simulink library "calcAeroCoeffs_cl"  (R2020a)
settings: Solver=VariableStepAuto  StartTime=0.0  StopTime=10.0  RelTol=1e-3
libraries: calculateCXorCZorCM_ul x3, calculateCYorCLorCN_ul x3
settings Model: Creator=Ayaz  LastModifiedBy=Ayaz

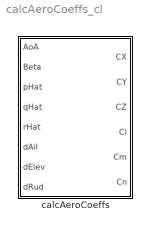
== system calcAeroCoeffs_cl ==
  calcAeroCoeffs : Subsystem  mask{C_X_AoA_coeffs=[8.32,0], C_X_qHat_coeffs=[4.41,-.6], C_X_dElev_coeffs=[0.11,-.01], C_X_0=0.46, C_Y_Beta_coeffs=-0.19, C_Y_pHat_coeffs=-0.1, C_Y_rHat_coeffs=[0.14,0.17], C_Y_dAil_coeffs=-0.05, C_Y_dRud_coeffs=0.1, C_Z_AoA_coeffs=[10.2,1.23,0], C_Z_qHat_coeffs=[6.15,0.13,-7.56], C_Z_dElev_coeffs=[0.29,0,-0.32], C_Z_0=-5.4, C_l_Beta_coeffs=-0.06, C_l_pHat_coeffs=-0.56, C_l_rHat_coeffs=[0.65,0.18], C_l_dAil_coeffs=[0.04,-0.25], C_l_dRud_coeffs=0, C_m_AoA_coeffs=[0.21,0], C_m_qHat_coeffs=[5.29,0,-11.30], C_m_dElev_coeffs=-1.02, C_m_0=-0.32, C_n_Beta_coeffs=[-0.09,0.06], C_n_pHat_coeffs=[-0.91,-0.06], C_n_rHat_coeffs=-0.05, C_n_dAil_coeffs=[-0.12,0.02], C_n_dRud_coeffs=-.04}
      mask prompts: C_X_AoA_coeffs "C_X_AoA polynomial coefficients (c0,c1,c2):"; C_X_qHat_coeffs "C_X_qHat polynomial coefficients (c0,c1,c2):"; C_X_dElev_coeffs "C_X_dElev polynomial coefficients (c0,c1,c2):"; C_X_0 "C_X_0 value"; C_Y_Beta_coeffs "C_Y_Beta polynomial coefficients (c0,c1,c2):"; C_Y_pHat_coeffs "C_Y_pHat polynomial coefficients (c0,c1,c2):"; C_Y_rHat_coeffs "C_Y_rHat polynomial coefficients (c0,c1,c2):"; C_Y_dAil_coeffs "C_Y_dAil polynomial coefficients (c0,c1,c2):"; C_Y_dRud_coeffs "C_Y_dRud polynomial coefficients (c0,c1,c2):"; C_Z_AoA_coeffs "C_Z_AoA polynomial coefficients (c0,c1,c2):"; C_Z_qHat_coeffs "C_Z_qHat polynomial coefficients (c0,c1,c2):"; C_Z_dElev_coeffs "C_Z_dElev polynomial coefficients (c0,c1,c2):"; C_Z_0 "C_Z_0 value"; C_l_Beta_coeffs "C_l_Beta polynomial coefficients (c0,c1,c2):"; C_l_pHat_coeffs "C_l_pHat polynomial coefficients (c0,c1,c2):"; C_l_rHat_coeffs "C_l_rHat polynomial coefficients (c0,c1,c2):"; C_l_dAil_coeffs "C_l_dAil polynomial coefficients (c0,c1,c2):"; C_l_dRud_coeffs "C_l_dRud polynomial coefficients (c0,c1,c2):"; C_m_AoA_coeffs "C_m_AoA polynomial coefficients (c0,c1,c2):"; C_m_qHat_coeffs "C_m_qHat polynomial coefficients (c0,c1,c2):"; C_m_dElev_coeffs "C_m_dElev polynomial coefficients (c0,c1,c2):"; C_m_0 "C_m_0 value"; C_n_Beta_coeffs "C_n_Beta polynomial coefficients (c0,c1,c2):"; C_n_pHat_coeffs "C_n_pHat polynomial coefficients (c0,c1,c2):"; C_n_rHat_coeffs "C_n_rHat polynomial coefficients (c0,c1,c2):"; C_n_dAil_coeffs "C_n_dAil polynomial coefficients (c0,c1,c2):"; C_n_dRud_coeffs "C_n_dRud polynomial coefficients (c0,c1,c2):"
      mask TypeOptions C_X_AoA_coeffs: calcCX/C_i_AoA_coeffs
      mask TypeOptions C_X_qHat_coeffs: calcCX/C_i_qHat_coeffs
      mask TypeOptions C_X_dElev_coeffs: calcCX/C_i_dElev_coeffs
      mask TypeOptions C_X_0: calcCX/C_i_0
      mask TypeOptions C_Y_Beta_coeffs: calcCY/C_i_Beta_coeffs
      mask TypeOptions C_Y_pHat_coeffs: calcCY/C_i_pHat_coeffs
      mask TypeOptions C_Y_rHat_coeffs: calcCY/C_i_rHat_coeffs
      mask TypeOptions C_Y_dAil_coeffs: calcCY/C_i_dAil_coeffs
      mask TypeOptions C_Y_dRud_coeffs: calcCY/C_i_dRud_coeffs
      mask TypeOptions C_Z_AoA_coeffs: calcCZ/C_i_AoA_coeffs
      mask TypeOptions C_Z_qHat_coeffs: calcCZ/C_i_qHat_coeffs
      mask TypeOptions C_Z_dElev_coeffs: calcCZ/C_i_dElev_coeffs
      mask TypeOptions C_Z_0: calcCZ/C_i_0
      mask TypeOptions C_l_Beta_coeffs: calcCl/C_i_Beta_coeffs
      mask TypeOptions C_l_pHat_coeffs: calcCl/C_i_pHat_coeffs
      mask TypeOptions C_l_rHat_coeffs: calcCl/C_i_rHat_coeffs
      mask TypeOptions C_l_dAil_coeffs: calcCl/C_i_dAil_coeffs
      mask TypeOptions C_l_dRud_coeffs: calcCl/C_i_dRud_coeffs
      mask TypeOptions C_m_AoA_coeffs: calcCm/C_i_AoA_coeffs
      mask TypeOptions C_m_qHat_coeffs: calcCm/C_i_qHat_coeffs
      mask TypeOptions C_m_dElev_coeffs: calcCm/C_i_dElev_coeffs
      mask TypeOptions C_m_0: calcCm/C_i_0
      mask TypeOptions C_n_Beta_coeffs: calcCn/C_i_Beta_coeffs
      mask TypeOptions C_n_pHat_coeffs: calcCn/C_i_pHat_coeffs
      mask TypeOptions C_n_rHat_coeffs: calcCn/C_i_rHat_coeffs
      mask TypeOptions C_n_dAil_coeffs: calcCn/C_i_dAil_coeffs
      mask TypeOptions C_n_dRud_coeffs: calcCn/C_i_dRud_coeffs
      mask DialogControl Container5 Prompt: Force CX coefficients
      mask DialogControl Container3 Prompt: Force CY coefficients
      mask DialogControl Container4 Prompt: Force CZ coefficients
      mask DialogControl Container6 Prompt: Moment Cl coefficients
      mask DialogControl Container7 Prompt: Moment Cm coefficients
      mask DialogControl Container8 Prompt: Moment Cn coefficients

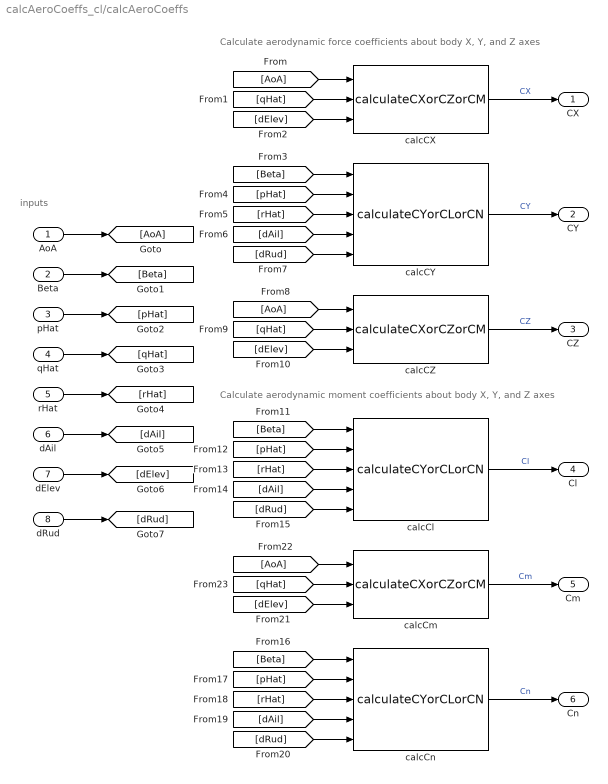
== system calcAeroCoeffs_cl/calcAeroCoeffs ==
  note: Calculate aerodynamic moment coefficients about body X, Y, and Z axes
  note: Calculate aerodynamic force coefficients about body X, Y, and Z axes
  note: inputs
  AoA : Inport
  Beta : Inport  Port=2
  pHat : Inport  Port=3
  qHat : Inport  Port=4
  rHat : Inport  Port=5
  dAil : Inport  Port=6
  dElev : Inport  Port=7
  dRud : Inport  Port=8
  calcCX : calculateCXorCZorCM_ul/calculateCXorCZorCM  C_i_AoA_coeffs=C_X_AoA_coeffs  C_i_qHat_coeffs=C_X_qHat_coeffs  C_i_dElev_coeffs=C_X_dElev_coeffs  C_i_0=C_X_0
  calcCY : calculateCYorCLorCN_ul/calculateCYorCLorCN  C_i_Beta_coeffs=C_Y_Beta_coeffs  C_i_pHat_coeffs=C_Y_pHat_coeffs  C_i_rHat_coeffs=C_Y_rHat_coeffs  C_i_dAil_coeffs=C_Y_dAil_coeffs  C_i_dRud_coeffs=C_Y_dRud_coeffs
  calcCZ : calculateCXorCZorCM_ul/calculateCXorCZorCM  C_i_AoA_coeffs=C_Z_AoA_coeffs  C_i_qHat_coeffs=C_Z_qHat_coeffs  C_i_dElev_coeffs=C_Z_dElev_coeffs  C_i_0=C_Z_0
  calcCl : calculateCYorCLorCN_ul/calculateCYorCLorCN  C_i_Beta_coeffs=C_l_Beta_coeffs  C_i_pHat_coeffs=C_l_pHat_coeffs  C_i_rHat_coeffs=C_l_rHat_coeffs  C_i_dAil_coeffs=C_l_dAil_coeffs  C_i_dRud_coeffs=C_l_dRud_coeffs
  calcCm : calculateCXorCZorCM_ul/calculateCXorCZorCM  C_i_AoA_coeffs=C_m_AoA_coeffs  C_i_qHat_coeffs=C_m_qHat_coeffs  C_i_dElev_coeffs=C_m_dElev_coeffs  C_i_0=C_m_0
  calcCn : calculateCYorCLorCN_ul/calculateCYorCLorCN  C_i_Beta_coeffs=C_n_Beta_coeffs  C_i_pHat_coeffs=C_n_pHat_coeffs  C_i_rHat_coeffs=C_n_rHat_coeffs  C_i_dAil_coeffs=C_n_dAil_coeffs  C_i_dRud_coeffs=C_n_dRud_coeffs
  CX : Outport
  CY : Outport  Port=2
  CZ : Outport  Port=3
  Cl : Outport  Port=4
  Cm : Outport  Port=5
  Cn : Outport  Port=6
  wires:
  calcCX/1 -> CX/1  "CX"
  calcCY/1 -> CY/1  "CY"
  calcCZ/1 -> CZ/1  "CZ"
  calcCl/1 -> Cl/1  "Cl"
  calcCm/1 -> Cm/1  "Cm"
  calcCn/1 -> Cn/1  "Cn"
  AoA/1 -> [AoA]
  Beta/1 -> [Beta]
  pHat/1 -> [pHat]
  qHat/1 -> [qHat]
  rHat/1 -> [rHat]
  dAil/1 -> [dAil]
  dElev/1 -> [dElev]
  dRud/1 -> [dRud]
  [AoA] -> calcCX/1
  [qHat] -> calcCX/2
  [dElev] -> calcCX/3
  [Beta] -> calcCY/1
  [pHat] -> calcCY/2
  [rHat] -> calcCY/3
  [dAil] -> calcCY/4
  [dRud] -> calcCY/5
  [dElev] -> calcCZ/3
  [AoA] -> calcCZ/1
  [qHat] -> calcCZ/2
  [pHat] -> calcCl/2
  [rHat] -> calcCl/3
  [Beta] -> calcCl/1
  [dRud] -> calcCl/5
  [dAil] -> calcCl/4
  [pHat] -> calcCn/2
  [rHat] -> calcCn/3
  [Beta] -> calcCn/1
  [dRud] -> calcCn/5
  [dAil] -> calcCn/4
  [qHat] -> calcCm/2
  [dElev] -> calcCm/3
  [AoA] -> calcCm/1
